simulink model "OFDM_Tx_Rx_InterpDec"  (R2020a)
settings: Solver=FixedStepDiscrete  StartTime=0.0  StopTime=inf  RelTol=1e-3
InitFcn:
  | % Set parameters
  | fs = 200e3;
  | 
  | % Load all required variables
  | load('read_addr_data');
  | load('read_addr_cp');
  | load('read_addr_pream');
  | load('read_addr_rx');
  | load('pilot');
  | load('LTSfreq');
  | load('STSfreq');
  | load('LTSread');
  | load('STSread');
  | load('bpsk');
  | load('qpsk');
  | load('qam16');
values from neighbouring files (symbols this model uses):
  bpsk = [0 0 1 1 1 1 0 0 1 0 1 0 ... (48 elements, 48x1)]    [bpsk.mat]
  qam16 = [12 5 10 3 14 8 1 10 8 7 2 13 ... (48 elements, 48x1)]    [qam16.mat]
  qpsk = [1 2 1 2 2 2 3 1 1 3 1 0 ... (48 elements, 48x1)]    [qpsk.mat]
  STSfreq = [0 0 0 0 0 0 0 0 1 0 0 0 ... (64 elements, 1x64)]    [STSfreq.mat]
undefined symbols (not defined in the file or in its folder): data3, designMultirateFIR, LTSfreq, LTSread, pilot, read_addr_cp, read_addr_data, read_addr_pream, read_addr_rx, STSread
libraries: hdlsllib x58, simulink x42, dspmlti4 x8, dsphdlxfrm x2, dsphdlmathfun x2, dsphdlsigops x1
(part 5 of 5)

== system OFDM_Tx_Rx_InterpDec/OFDMRx/Synchronisation/FineTimingSynch/MatchedFilter/Subsystem59 ==
  MatchedIn : Inport
  Add : Sum  OutDataTypeStr=fixdt(1,18,14)
  Add1 : Sum  Inputs=+-  OutDataTypeStr=fixdt(1,18,14)
  Complex to Real-Imag : ComplexToRealImag
  Real-Imag to Complex : RealImagToComplex
  Out1 : Outport
  wires:
  Real-Imag to Complex/1 -> Out1/1
  MatchedIn/1 -> Complex to Real-Imag/1
  Complex to Real-Imag/1 -> Add/1, Add1/2
  Add1/1 -> Real-Imag to Complex/2
  Add/1 -> Real-Imag to Complex/1
  Complex to Real-Imag/2 -> Add/2, Add1/1

== system OFDM_Tx_Rx_InterpDec/OFDMRx/Synchronisation/FineTimingSynch/MatchedFilter/Subsystem6 ==
  MatchedIn : Inport
  Add : Sum  OutDataTypeStr=fixdt(1,18,14)
  Add1 : Sum  Inputs=+-  OutDataTypeStr=fixdt(1,18,14)
  Complex to Real-Imag : ComplexToRealImag
  Real-Imag to Complex : RealImagToComplex
  Unary Minus : UnaryMinus
  Out1 : Outport
  wires:
  Real-Imag to Complex/1 -> Out1/1
  MatchedIn/1 -> Complex to Real-Imag/1
  Add1/1 -> Real-Imag to Complex/1
  Complex to Real-Imag/2 -> Add/2, Add1/1
  Complex to Real-Imag/1 -> Add/1, Add1/2
  Add/1 -> Unary Minus/1
  Unary Minus/1 -> Real-Imag to Complex/2

== system OFDM_Tx_Rx_InterpDec/OFDMRx/Synchronisation/FineTimingSynch/MatchedFilter/Subsystem60 ==
  MatchedIn : Inport
  Add : Sum  OutDataTypeStr=fixdt(1,18,14)
  Add1 : Sum  Inputs=+-  OutDataTypeStr=fixdt(1,18,14)
  Complex to Real-Imag : ComplexToRealImag
  Real-Imag to Complex : RealImagToComplex
  Out1 : Outport
  wires:
  Complex to Real-Imag/2 -> Add1/1, Add/2
  Add/1 -> Real-Imag to Complex/1
  Add1/1 -> Real-Imag to Complex/2
  Complex to Real-Imag/1 -> Add1/2, Add/1
  MatchedIn/1 -> Complex to Real-Imag/1
  Real-Imag to Complex/1 -> Out1/1

== system OFDM_Tx_Rx_InterpDec/OFDMRx/Synchronisation/FineTimingSynch/MatchedFilter/Subsystem61 ==
  MatchedIn : Inport
  Add : Sum  OutDataTypeStr=fixdt(1,18,14)
  Add1 : Sum  Inputs=+-  OutDataTypeStr=fixdt(1,18,14)
  Complex to Real-Imag : ComplexToRealImag
  Real-Imag to Complex : RealImagToComplex
  Out1 : Outport
  wires:
  Add/1 -> Real-Imag to Complex/2
  Add1/1 -> Real-Imag to Complex/1
  Complex to Real-Imag/2 -> Add/2, Add1/2
  Complex to Real-Imag/1 -> Add/1, Add1/1
  MatchedIn/1 -> Complex to Real-Imag/1
  Real-Imag to Complex/1 -> Out1/1

== system OFDM_Tx_Rx_InterpDec/OFDMRx/Synchronisation/FineTimingSynch/MatchedFilter/Subsystem62 ==
  MatchedIn : Inport
  Add : Sum  OutDataTypeStr=fixdt(1,18,14)
  Add1 : Sum  Inputs=+-  OutDataTypeStr=fixdt(1,18,14)
  Complex to Real-Imag : ComplexToRealImag
  Real-Imag to Complex : RealImagToComplex
  Unary Minus : UnaryMinus
  Out1 : Outport
  wires:
  Unary Minus/1 -> Real-Imag to Complex/1
  Real-Imag to Complex/1 -> Out1/1
  MatchedIn/1 -> Complex to Real-Imag/1
  Complex to Real-Imag/1 -> Add/1, Add1/1
  Add1/1 -> Real-Imag to Complex/2
  Add/1 -> Unary Minus/1
  Complex to Real-Imag/2 -> Add/2, Add1/2

== system OFDM_Tx_Rx_InterpDec/OFDMRx/Synchronisation/FineTimingSynch/MatchedFilter/Subsystem63 ==
  MatchedIn : Inport
  Add : Sum  OutDataTypeStr=fixdt(1,18,14)
  Add1 : Sum  Inputs=+-  OutDataTypeStr=fixdt(1,18,14)
  Complex to Real-Imag : ComplexToRealImag
  Real-Imag to Complex : RealImagToComplex
  Unary Minus : UnaryMinus
  Out1 : Outport
  wires:
  Real-Imag to Complex/1 -> Out1/1
  MatchedIn/1 -> Complex to Real-Imag/1
  Add1/1 -> Real-Imag to Complex/1
  Complex to Real-Imag/2 -> Add/2, Add1/1
  Complex to Real-Imag/1 -> Add/1, Add1/2
  Add/1 -> Unary Minus/1
  Unary Minus/1 -> Real-Imag to Complex/2

== system OFDM_Tx_Rx_InterpDec/OFDMRx/Synchronisation/FineTimingSynch/MatchedFilter/Subsystem7 ==
  MatchedIn : Inport
  Add : Sum  OutDataTypeStr=fixdt(1,18,14)
  Add1 : Sum  Inputs=+-  OutDataTypeStr=fixdt(1,18,14)
  Complex to Real-Imag : ComplexToRealImag
  Real-Imag to Complex : RealImagToComplex
  Out1 : Outport
  wires:
  Real-Imag to Complex/1 -> Out1/1
  MatchedIn/1 -> Complex to Real-Imag/1
  Complex to Real-Imag/1 -> Add/1, Add1/2
  Add1/1 -> Real-Imag to Complex/2
  Add/1 -> Real-Imag to Complex/1
  Complex to Real-Imag/2 -> Add/2, Add1/1

== system OFDM_Tx_Rx_InterpDec/OFDMRx/Synchronisation/FineTimingSynch/MatchedFilter/Subsystem8 ==
  MatchedIn : Inport
  Add : Sum  OutDataTypeStr=fixdt(1,18,14)
  Add1 : Sum  Inputs=+-  OutDataTypeStr=fixdt(1,18,14)
  Complex to Real-Imag : ComplexToRealImag
  Real-Imag to Complex : RealImagToComplex
  Out1 : Outport
  wires:
  Add/1 -> Real-Imag to Complex/2
  Add1/1 -> Real-Imag to Complex/1
  Complex to Real-Imag/2 -> Add/2, Add1/2
  Complex to Real-Imag/1 -> Add/1, Add1/1
  MatchedIn/1 -> Complex to Real-Imag/1
  Real-Imag to Complex/1 -> Out1/1

== system OFDM_Tx_Rx_InterpDec/OFDMRx/Synchronisation/FineTimingSynch/MatchedFilter/Subsystem9 ==
  MatchedIn : Inport
  Add : Sum  OutDataTypeStr=fixdt(1,18,14)
  Add1 : Sum  Inputs=+-  OutDataTypeStr=fixdt(1,18,14)
  Complex to Real-Imag : ComplexToRealImag
  Real-Imag to Complex : RealImagToComplex
  Out1 : Outport
  wires:
  Real-Imag to Complex/1 -> Out1/1
  MatchedIn/1 -> Complex to Real-Imag/1
  Complex to Real-Imag/1 -> Add/1, Add1/2
  Add1/1 -> Real-Imag to Complex/2
  Add/1 -> Real-Imag to Complex/1
  Complex to Real-Imag/2 -> Add/2, Add1/1

== system OFDM_Tx_Rx_InterpDec/OFDMRx/Synchronisation/CoarseTimingSynch/CoarseTimeStrobeGen/LocalSearchCounter/RsingEdge ==
  In1 : Inport
  Delay : Delay  DelayLength=1
  Relational Operator : RelationalOperator  Operator=>  OutDataTypeStr=boolean  RndMeth=Nearest
  Out1 : Outport  VectorParamsAs1DForOutWhenUnconnected=off
  wires:
  Relational Operator/1 -> Out1/1
  Delay/1 -> Relational Operator/2
  In1/1 -> Delay/1, Relational Operator/1

== matlab function OFDM_Tx_Rx_InterpDec/OFDMTx/DataGenerator/Data Multiplexer ==
  data: symbols input; dataready input; data output; pilots input; pval input; sts input; stsval input; lts input; ltsval input
function data  = dataMux(symbols,dataready,pilots,pval,sts,stsval,lts,ltsval)
% Data multiplexer 
if (pval == true)
    data = pilots; 
elseif (stsval == true)
    data = sts; 
elseif (ltsval == true)
    data = lts; 
elseif (dataready == true) 
    data = symbols;
else 
    data = fi(complex(0),1,16,14);
end

== matlab function OFDM_Tx_Rx_InterpDec/OFDMTx/SCMapper/Mux2 ==
  data: preamb input; preambVal input; dataOut output; data input; dataVal input
function dataOut = mux(preamb,preambVal,data,dataVal)

if (preambVal == true)
    dataOut = preamb; 
elseif (dataVal == true)
    dataOut = data; 
else 
    dataOut = fi(complex(0),1,16,14);
end

== matlab function OFDM_Tx_Rx_InterpDec/OFDMTx/CPAdd/Mux2 ==
  data: sts input; stsval input; lts input; ltsval input; dataOut output; data input; dataval input
function dataOut = mux(sts,stsval,lts,ltsval,data,dataval)

if (stsval == true)
    dataOut = sts; 
elseif (ltsval == true)
    dataOut = lts; 
elseif (dataval == true) 
    dataOut = data; 
else 
    dataOut = fi(complex(0),1,16,14);
end

== matlab function OFDM_Tx_Rx_InterpDec/OFDMRx/PhaseTracking/CordicRotate/QMAP/QUAD_MAP1 ==
  data: xin input; xout output; yout output; yin input; ctrl input
function [xout,yout] = fcn(xin,yin,ctrl)
% Process to perform final rotation 
% by pi/2 if the original angle was 
% in 3rd or 4th quadrants    
if ctrl == 0
    % 1st or 2nd quadrants 
    xout = fi(xin,1,21,15);  
    yout = fi(yin,1,21,15);  
elseif ctrl == 1
    % 3rd quadrant (rotate pi/2 clockwise)
    xout = fi(yin,1,21,15); 
    yout = fi(-xin,1,21,15); 
elseif ctrl == 2
    % 4th quadrant (rotate pi/2 anti-clockwise) 
    xout = fi(-yin,1,21,15); 
    yout = fi(xin,1,21,15); 
else 
    % others clause
    xout = fi(xin,1,21,15); 
    yout = fi(yin,1,21,15); 
end

== matlab function OFDM_Tx_Rx_InterpDec/OFDMRx/PhaseTracking/CordicRotate/QUAD_MAP/QUAD_DETERM1 ==
  data: ang_in input; ang_out output; QUAD output
function [ang_out,QUAD] = fcn(ang_in)
% Process to determine quadrant and 
% shift into region -pi/2 to pi/2 if 
% not already there 
v = fi(pi,1,23,20);
x = fi(-pi,1,23,20); 
y = fi(-pi/2,1,23,20); 
z = fi(pi/2,1,23,20);

% Determine quadrant 
if ((ang_in >= y) && (ang_in <= z))
    QUAD = fi(0,0,2,0); % Quads 1 or 2
elseif ((ang_in < y) && (ang_in >= x))
    QUAD = fi(1,0,2,0); % Quad 3
elseif ((ang_in > z) && (ang_in <= v))
    QUAD = fi(2,0,2,0); % Quad 4
else 
    % others clause
    QUAD = fi(0,0,2,0);
end 

% Determine whether we need to add or subtract pi/2 
% based on quadrant location
switch(QUAD) 
    
    case 0 
        % Angle stays the same 
        ang_out = fi(ang_in, 1, 23, 20); 
    case 1
        % pi/2 is added to angle (anti-clockwise)
        ang_out = fi(ang_in + z, 1, 23, 20); 
    case 2
        % pi/2 is subtracted from angle (clockwise)
        ang_out = fi(ang_in - z, 1, 23, 20); 
    otherwise
        % others clause make output angle 
        % equal to input angle  
        ang_out = fi(ang_in, 1, 23, 20); 
end
